simulink model "Trotter_nonsymbolic_VarPhiD"  (R2024a)
settings: Solver=daessc  StartTime=0.0  StopTime=5  FixedStep=1e-5  MaxStep=1e-3  RelTol=1e-5  AbsTol=1e-5  EnableMultiTasking=on
values from neighbouring files (symbols this model uses):
  alpha0 = states{3}(indexVector{3})    [RunAllVPPTrials.m]    (also in SimulationConfig.m = 1.74532925199)
  Bground = 5e3    (= 5000)    [SimulationConfig.m]
  grav = -9.80665    [SimulationConfig.m]
  groundLx = 1000    [SimulationConfig.m]
  groundLy = 1000    [SimulationConfig.m]
  groundThickness = 0.1    [SimulationConfig.m]
  hipSwingStiffness = states{6}(indexVector{6})    [RunAllVPPTrials.m]    (also in SimulationConfig.m = 1000)
  Ka = states{7}(indexVector{7})    [RunAllVPPTrials.m]    (also in SimulationConfig.m = 500)
  Kground = 1e5    (= 100000)    [SimulationConfig.m]
  L1 = 1    [SimulationConfig.m]
  L2 = 1    [SimulationConfig.m]
  m1 = 0.001    [SimulationConfig.m]
  m2 = 0.001    [SimulationConfig.m]
  maxKgLimit = 40000    [SimulationConfig.m]
  mf = 0.001    [SimulationConfig.m]
  mHip = 10    [SimulationConfig.m]
  omega = (strideAngle*pi/180)*(2*hipFreq)    [RunAllVPPTrials.m]    (also in SimulationConfig.m = 2.79252680319)
  phi0 = acos((L1^2-L2^2-f2h0^2)/-(2*L2*f2h0))    [RunAllVPPTrials.m]    (also in SimulationConfig.m)
  rf = 0.05    [SimulationConfig.m]
  shouldIAdaptKp = 1    [RunAllVPPTrials.m]    (also in SimulationConfig.m)
  startingHipStiffness = 1000    [SimulationConfig.m]
  startupTime = 0    [SimulationConfig.m]
  strideAngle = states{4}(indexVector{4})    [RunAllVPPTrials.m]    (also in SimulationConfig.m = 40)
  torsoHeight = 0.2    [SimulationConfig.m]
  torsoLength = 2.5    [SimulationConfig.m]
  torsoWidth = 0.2    [SimulationConfig.m]
  y0 = f2h0*sin(beta0+pi/2)    [RunAllVPPTrials.m]    (also in SimulationConfig.m)
  yOffset = 0.1    [SimulationConfig.m]
undefined symbols (not defined in the file or in its folder): X, Y, Z
libraries: sm_lib x113, nesl_utility x88, Contact_Forces_Lib x16, simulink x8
(part 7 of 7)

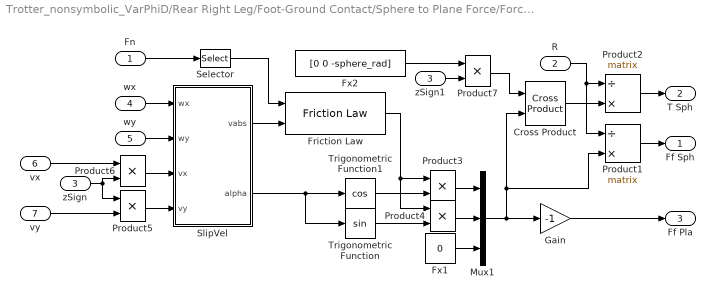
== system Trotter_nonsymbolic_VarPhiD/Rear Right Leg/Foot-Ground Contact/Sphere to Plane Force/Forces/Ff ==
  Fn : Inport
  R : Inport  Port=2
  zSign : Inport  Port=3
  wx : Inport  Port=4
  wy : Inport  Port=5
  vx : Inport  Port=6
  vy : Inport  Port=7
  Cross Product : Contact_Forces_Lib/Math/Cross Product  SystemSampleTime=-1  VariantActivationTime=update diagram  AllowFlexibleInterface=on  Latency=0  AutoFrameSizeCalculation=off
      settings: SourceProductName=Simscape Multibody Contact Forces Library
  Friction Law : Contact_Forces_Lib/Friction Law  SystemSampleTime=-1  LabelModeActiveChoice=Stick_Slip_C  VariantActivationTime=update diagram  AllowFlexibleInterface=on  Latency=0  AutoFrameSizeCalculation=off
      settings: SourceProductName=Simscape Multibody Contact Forces Library
  Fx1 : Constant  Value=0
  Fx2 : Constant  Value=[0 0 -sphere_rad]
  Gain : Gain  Gain=-1
  Mux1 : Mux  Inputs=3
  Product1 : Product  Inputs=/*  Multiplication=Matrix(*)
  Product2 : Product  Inputs=/*  Multiplication=Matrix(*)
  Product{3..7} (5 alike) : Product
  Selector : Selector  InputPortWidth=3  IndexOptions=Index vector (dialog)  Indices=3  OutputSizes=1
  SlipVel : Subsystem
  Trigonometric Function : Trigonometry
  Trigonometric Function1 : Trigonometry  Operator=cos
  zSign1 : InportShadow  Port=3
  Ff Sph : Outport  VectorParamsAs1DForOutWhenUnconnected=off
  T Sph : Outport  Port=2  VectorParamsAs1DForOutWhenUnconnected=off
  Ff Pla : Outport  Port=3  VectorParamsAs1DForOutWhenUnconnected=off
  wires:
  Product7/1 -> Cross Product/1
  zSign1/1 -> Product7/2
  Product6/1 -> SlipVel/3(vx)
  zSign/1 -> Product6/2, Product5/1
  Product5/1 -> SlipVel/4(vy)
  Fx2/1 -> Product7/1
  R/1 -> Product2/1, Product1/1
  Cross Product/1 -> Product2/2
  Product1/1 -> Ff Sph/1
  Mux1/1 -> Product1/2, Cross Product/2, Gain/1
  Product2/1 -> T Sph/1
  vy/1 -> Product5/2
  wy/1 -> SlipVel/2(wy)
  wx/1 -> SlipVel/1(wx)
  vx/1 -> Product6/1
  Trigonometric Function/1 -> Product4/2
  Fx1/1 -> Mux1/3
  Product3/1 -> Mux1/1
  Product4/1 -> Mux1/2
  Friction Law/1 -> Product4/1, Product3/1
  Selector/1 -> Friction Law/1
  SlipVel/1(vabs) -> Friction Law/2
  Trigonometric Function1/1 -> Product3/2
  SlipVel/2(alpha) -> Trigonometric Function1/1, Trigonometric Function/1
  Gain/1 -> Ff Pla/1
  Fn/1 -> Selector/1

== system Trotter_nonsymbolic_VarPhiD/Rear Right Leg/Foot-Ground Contact/Sphere to Plane Force/Forces/Fn ==
  R : Inport
  SprF : Inport  Port=2
  DamF : Inport  Port=3
  Fx : Constant  Value=0
  Gain : Gain  Gain=-1
  Mux : Mux  Inputs=3
  Product2 : Product  Inputs=/*  Multiplication=Matrix(*)
  Sum : Sum
  Fn : Outport  VectorParamsAs1DForOutWhenUnconnected=off
  FnF : Outport  Port=2  VectorParamsAs1DForOutWhenUnconnected=off
  FnB : Outport  Port=3  VectorParamsAs1DForOutWhenUnconnected=off
  wires:
  SprF/1 -> Sum/1
  DamF/1 -> Sum/2
  Sum/1 -> Mux/3, Fn/1
  Fx/1 -> Mux/2, Mux/1
  R/1 -> Product2/1
  Gain/1 -> FnB/1
  Product2/1 -> FnF/1
  Mux/1 -> Product2/2, Gain/1

== system Trotter_nonsymbolic_VarPhiD/Front Left Leg/Foot-Ground Contact/Sphere to Plane Force/Forces/Ff/SlipVel ==
  wx : Inport
  wy : Inport  Port=2
  vx : Inport  Port=3
  vy : Inport  Port=4
  Fx1 : Constant  Value=sphere_rad
  Math Function : Math  Operator=square  SignedPower=on
  Math Function1 : Math  Operator=square  SignedPower=on
  Product3 : Product
  Product4 : Product
  Sqrt : Sqrt
  Sum1 : Sum  Inputs=|++
  Sum2 : Sum  Inputs=|-+
  Sum3 : Sum  Inputs=|++
  Trigonometric Function : Trigonometry  Operator=atan2
  vabs : Outport  VectorParamsAs1DForOutWhenUnconnected=off
  alpha : Outport  Port=2  VectorParamsAs1DForOutWhenUnconnected=off
  wires:
  wx/1 -> Product3/1
  Product3/1 -> Sum1/1
  wy/1 -> Product4/2
  vx/1 -> Sum2/2
  Fx1/1 -> Product3/2, Product4/1
  vy/1 -> Sum1/2
  Product4/1 -> Sum2/1
  Trigonometric Function/1 -> alpha/1
  Sqrt/1 -> vabs/1
  Sum3/1 -> Sqrt/1
  Math Function/1 -> Sum3/1
  Math Function1/1 -> Sum3/2
  Sum1/1 -> Trigonometric Function/1, Math Function/1  "slipy"
  Sum2/1 -> Trigonometric Function/2, Math Function1/1  "slipx"

== system Trotter_nonsymbolic_VarPhiD/Front Right Leg/Foot-Ground Contact/Sphere to Plane Force/Forces/Ff/SlipVel ==
  wx : Inport
  wy : Inport  Port=2
  vx : Inport  Port=3
  vy : Inport  Port=4
  Fx1 : Constant  Value=sphere_rad
  Math Function : Math  Operator=square  SignedPower=on
  Math Function1 : Math  Operator=square  SignedPower=on
  Product3 : Product
  Product4 : Product
  Sqrt : Sqrt
  Sum1 : Sum  Inputs=|++
  Sum2 : Sum  Inputs=|-+
  Sum3 : Sum  Inputs=|++
  Trigonometric Function : Trigonometry  Operator=atan2
  vabs : Outport  VectorParamsAs1DForOutWhenUnconnected=off
  alpha : Outport  Port=2  VectorParamsAs1DForOutWhenUnconnected=off
  wires:
  wx/1 -> Product3/1
  Product3/1 -> Sum1/1
  wy/1 -> Product4/2
  vx/1 -> Sum2/2
  Fx1/1 -> Product3/2, Product4/1
  vy/1 -> Sum1/2
  Product4/1 -> Sum2/1
  Trigonometric Function/1 -> alpha/1
  Sqrt/1 -> vabs/1
  Sum3/1 -> Sqrt/1
  Math Function/1 -> Sum3/1
  Math Function1/1 -> Sum3/2
  Sum1/1 -> Trigonometric Function/1, Math Function/1  "slipy"
  Sum2/1 -> Trigonometric Function/2, Math Function1/1  "slipx"

== system Trotter_nonsymbolic_VarPhiD/Rear Left Leg/Foot-Ground Contact/Sphere to Plane Force/Forces/Ff/SlipVel ==
  wx : Inport
  wy : Inport  Port=2
  vx : Inport  Port=3
  vy : Inport  Port=4
  Fx1 : Constant  Value=sphere_rad
  Math Function : Math  Operator=square  SignedPower=on
  Math Function1 : Math  Operator=square  SignedPower=on
  Product3 : Product
  Product4 : Product
  Sqrt : Sqrt
  Sum1 : Sum  Inputs=|++
  Sum2 : Sum  Inputs=|-+
  Sum3 : Sum  Inputs=|++
  Trigonometric Function : Trigonometry  Operator=atan2
  vabs : Outport  VectorParamsAs1DForOutWhenUnconnected=off
  alpha : Outport  Port=2  VectorParamsAs1DForOutWhenUnconnected=off
  wires:
  wx/1 -> Product3/1
  Product3/1 -> Sum1/1
  wy/1 -> Product4/2
  vx/1 -> Sum2/2
  Fx1/1 -> Product3/2, Product4/1
  vy/1 -> Sum1/2
  Product4/1 -> Sum2/1
  Trigonometric Function/1 -> alpha/1
  Sqrt/1 -> vabs/1
  Sum3/1 -> Sqrt/1
  Math Function/1 -> Sum3/1
  Math Function1/1 -> Sum3/2
  Sum1/1 -> Trigonometric Function/1, Math Function/1  "slipy"
  Sum2/1 -> Trigonometric Function/2, Math Function1/1  "slipx"

== system Trotter_nonsymbolic_VarPhiD/Rear Right Leg/Foot-Ground Contact/Sphere to Plane Force/Forces/Ff/SlipVel ==
  wx : Inport
  wy : Inport  Port=2
  vx : Inport  Port=3
  vy : Inport  Port=4
  Fx1 : Constant  Value=sphere_rad
  Math Function : Math  Operator=square  SignedPower=on
  Math Function1 : Math  Operator=square  SignedPower=on
  Product3 : Product
  Product4 : Product
  Sqrt : Sqrt
  Sum1 : Sum  Inputs=|++
  Sum2 : Sum  Inputs=|-+
  Sum3 : Sum  Inputs=|++
  Trigonometric Function : Trigonometry  Operator=atan2
  vabs : Outport  VectorParamsAs1DForOutWhenUnconnected=off
  alpha : Outport  Port=2  VectorParamsAs1DForOutWhenUnconnected=off
  wires:
  wx/1 -> Product3/1
  Product3/1 -> Sum1/1
  wy/1 -> Product4/2
  vx/1 -> Sum2/2
  Fx1/1 -> Product3/2, Product4/1
  vy/1 -> Sum1/2
  Product4/1 -> Sum2/1
  Trigonometric Function/1 -> alpha/1
  Sqrt/1 -> vabs/1
  Sum3/1 -> Sqrt/1
  Math Function/1 -> Sum3/1
  Math Function1/1 -> Sum3/2
  Sum1/1 -> Trigonometric Function/1, Math Function/1  "slipy"
  Sum2/1 -> Trigonometric Function/2, Math Function1/1  "slipx"

== matlab function Trotter_nonsymbolic_VarPhiD/Left Side Trajectory Generator ==
  data: t input; y_out output; omega parameter; strideAngle parameter; tau output
function [y_out,tau] = fcn(t, omega, strideAngle)
r = (strideAngle*pi/180)/2;% +/- rad (total leg sweep angle is 2*strideAngle)
T = 4*r/omega;
% tau = mod(t+T/4,T)/T; % This starts the trajectory as if the leg is vertically downward during retraction
tau = mod(t+T/2,T)/T; % This starts the trajectory as if the leg is in a backward position a little before protraction begins
% tau = mod(t,T)/T;       % This starts the trajectory as if the leg is in a forward position, right as retraction begins
if tau<0.5
    y_out = r-omega*T*tau;
    dy_out = -omega*T;
else
    y_out = -r - omega*T*(tau-0.5)...
        +(24*r+6*omega*T)*(tau-0.5)^2+(-32*r-8*omega*T)*(tau-0.5)^3;
    dy_out = r*(-96*tau^2+144*tau-48)+(-24*tau^2+36*tau-13)*T*omega;
end

== matlab function Trotter_nonsymbolic_VarPhiD/Front Left Leg/Toe lift ==
  data: tau input; y output; L1 parameter
function y = fcn(tau, L1)
% A = 8*L1;
% y = A*(u-0.75)^2+(1/4)*L1;
% y = min(y,3*L1/4);

a0 = 1/2;
a1 = 0;
a2 = -12;
a3 = 16;
if(tau>=0.5)
    y = L1*(abs((a0+a1*(tau-0.5)+a2*(tau-0.5).^2+a3*(tau-0.5).^3))+0.25);
else
    y = L1*0.75;
end

== matlab function Trotter_nonsymbolic_VarPhiD/Right Side Trajectory Generator ==
  data: t input; y_out output; omega parameter; strideAngle parameter; tau output
function [y_out,tau] = fcn(t, omega, strideAngle)
r = (strideAngle*pi/180)/2;% +/- rad (total leg sweep angle is 2*strideAngle)
T = 4*r/omega;
% tau = mod(t+T/4,T)/T; % This starts the trajectory as if the leg is vertically downward during retraction
% tau = mod(t+T/2,T)/T; % This starts the trajectory as if the leg is in a backward position a little before protraction begins
tau = mod(t,T)/T;       % This starts the trajectory as if the leg is in a forward position, right as retraction begins
if tau<0.5
    y_out = r-omega*T*tau;
    dy_out = -omega*T;
else
    y_out = -r - omega*T*(tau-0.5)...
        +(24*r+6*omega*T)*(tau-0.5)^2+(-32*r-8*omega*T)*(tau-0.5)^3;
    dy_out = r*(-96*tau^2+144*tau-48)+(-24*tau^2+36*tau-13)*T*omega;
end

== matlab function Trotter_nonsymbolic_VarPhiD/Rear Left Leg/Toe lift ==
  data: tau input; y output; L1 parameter
function y = fcn(tau, L1)
% A = 8*L1;
% y = A*(u-0.75)^2+(1/4)*L1;
% y = min(y,3*L1/4);

a0 = 1/2;
a1 = 0;
a2 = -12;
a3 = 16;
if(tau>=0.5)
    y = L1*(abs((a0+a1*(tau-0.5)+a2*(tau-0.5).^2+a3*(tau-0.5).^3))+0.25);
else
    y = L1*0.75;
end

== matlab function Trotter_nonsymbolic_VarPhiD/Front Right Leg/MATLAB Function ==
  data: tau input; y output; L1 parameter
function y = fcn(tau, L1)
% A = 8*L1;
% y = A*(u-0.75)^2+(1/4)*L1;
% y = min(y,3*L1/4);

a0 = 1/2;
a1 = 0;
a2 = -12;
a3 = 16;
if(tau>=0.5)
    y = L1*(abs((a0+a1*(tau-0.5)+a2*(tau-0.5).^2+a3*(tau-0.5).^3))+0.25);
else
    y = L1*0.75;
end

== matlab function Trotter_nonsymbolic_VarPhiD/Front Left Shoulder Joint/Calculate Kg Nonsymbolic ==
  data: time input; phiD input; f2hX input; f2hY input; gammaDesired input; gc input; deltaGamma input; tauHip output; Kout output; startingHipStiffness parameter; hipSwingStiffness parameter; startupTime parameter; shouldIAdaptKp parameter; L1 parameter; L2 parameter; alpha0 parameter; Ka parameter; maxKgLimit parameter
function [tauHip,Kout]  = fcn(time, phiD, f2hX, f2hY, gammaDesired, gc, deltaGamma, startingHipStiffness, hipSwingStiffness, startupTime, shouldIAdaptKp, L1, L2, alpha0, Ka, maxKgLimit)
persistent time_old;
if isempty(time_old)
    time_old = 0;
end
persistent Kg_pers;
if isempty(Kg_pers)
    Kg_pers = 1000;
end

if shouldIAdaptKp==1
    if time>startupTime
        if gc>0
            if time-time_old>=0.001
                x = f2hX;
                y = f2hY;
                gamma0 = gammaDesired+pi/2;
                thetad = phiD;
                Kg_pers = -((Ka*y*(alpha0 + acos((0.5000*L1^2 + 0.5000*L2^2 - 0.5000*x^2 - 0.5000*y^2)/(L1*L2)) - pi))/(L1*L2*(1 - (0.2500*(L1^2 + L2^2 - x^2 - y^2)^2)/(L1^2*L2^2))^0.5000) - (Ka*x*tan(thetad)*(alpha0 + acos((0.5000*L1^2 + 0.5000*L2^2 - 0.5000*x^2 - 0.5000*y^2)/(L1*L2)) - pi))/(L1*L2*(1 - (0.2500*(L1^2 + L2^2 - x^2 - y^2)^2)/(L1^2*L2^2))^0.5000))/((acos((- 0.5000*L1^2 + 0.5000*L2^2 + 0.5000*x^2 + 0.5000*y^2)/(L2*(x^2 + y^2)^0.5000)) + atan2(1*y, x) - gamma0)*(tan(thetad)*((x/(L2*(x^2 + y^2)^0.5000) - (0.5000*x*(- L1^2 + L2^2 + x^2 + y^2))/(L2*(x^2 + y^2)^1.5000))/(1 - (0.2500*(- L1^2 + L2^2 + x^2 + y^2)^2)/(L2^2*(x^2 + y^2)))^0.5000 + y/(x^2 + y^2)) - (y/(L2*(x^2 + y^2)^0.5000) - (0.5000*y*(- L1^2 + L2^2 + x^2 + y^2))/(L2*(x^2 + y^2)^1.5000))/(1 - (0.2500*(- L1^2 + L2^2 + x^2 + y^2)^2)/(L2^2*(x^2 + y^2)))^0.5000 + x/(x^2 + y^2)));
                if ~isreal(Kg_pers)
                    Kg_pers=60;
                end
                Kg_pers = min(max(100,Kg_pers),maxKgLimit);
                time_old = time;
            end
        else
            Kg_pers = hipSwingStiffness;
        end
    else
        Kg_pers = startingHipStiffness;
    end
else
    Kg_pers = hipSwingStiffness;
end
tauHip = Kg_pers*deltaGamma;
Kout = Kg_pers;

% I added pi/2 to gammaDesired because the simulation has gamm=0deg as
% vertical but the matrix calculations and derivations used gamma=0deg as
% horizontal.

== matlab function Trotter_nonsymbolic_VarPhiD/Rear Left Hip Joint/Calculate Kg Nonsymbolic ==
  data: time input; phiD input; f2hX input; f2hY input; gammaDesired input; gc input; deltaGamma input; tauHip output; Kout output; startingHipStiffness parameter; hipSwingStiffness parameter; startupTime parameter; shouldIAdaptKp parameter; L1 parameter; L2 parameter; alpha0 parameter; Ka parameter; maxKgLimit parameter
function [tauHip,Kout]  = fcn(time, phiD, f2hX, f2hY, gammaDesired, gc, deltaGamma, startingHipStiffness, hipSwingStiffness, startupTime, shouldIAdaptKp, L1, L2, alpha0, Ka, maxKgLimit)
persistent time_old;
if isempty(time_old)
    time_old = 0;
end
persistent Kg_pers;
if isempty(Kg_pers)
    Kg_pers = 1000;
end

if shouldIAdaptKp==1
    if time>startupTime
        if gc>0
            if time-time_old>=0.001
                x = f2hX;
                y = f2hY;
                gamma0 = gammaDesired+pi/2;
                thetad = phiD;
                Kg_pers = -((Ka*y*(alpha0 + acos((0.5000*L1^2 + 0.5000*L2^2 - 0.5000*x^2 - 0.5000*y^2)/(L1*L2)) - pi))/(L1*L2*(1 - (0.2500*(L1^2 + L2^2 - x^2 - y^2)^2)/(L1^2*L2^2))^0.5000) - (Ka*x*tan(thetad)*(alpha0 + acos((0.5000*L1^2 + 0.5000*L2^2 - 0.5000*x^2 - 0.5000*y^2)/(L1*L2)) - pi))/(L1*L2*(1 - (0.2500*(L1^2 + L2^2 - x^2 - y^2)^2)/(L1^2*L2^2))^0.5000))/((acos((- 0.5000*L1^2 + 0.5000*L2^2 + 0.5000*x^2 + 0.5000*y^2)/(L2*(x^2 + y^2)^0.5000)) + atan2(1*y, x) - gamma0)*(tan(thetad)*((x/(L2*(x^2 + y^2)^0.5000) - (0.5000*x*(- L1^2 + L2^2 + x^2 + y^2))/(L2*(x^2 + y^2)^1.5000))/(1 - (0.2500*(- L1^2 + L2^2 + x^2 + y^2)^2)/(L2^2*(x^2 + y^2)))^0.5000 + y/(x^2 + y^2)) - (y/(L2*(x^2 + y^2)^0.5000) - (0.5000*y*(- L1^2 + L2^2 + x^2 + y^2))/(L2*(x^2 + y^2)^1.5000))/(1 - (0.2500*(- L1^2 + L2^2 + x^2 + y^2)^2)/(L2^2*(x^2 + y^2)))^0.5000 + x/(x^2 + y^2)));
                if ~isreal(Kg_pers)
                    Kg_pers=60;
                end
                Kg_pers = min(max(100,Kg_pers),maxKgLimit);
                time_old = time;
            end
        else
            Kg_pers = hipSwingStiffness;
        end
    else
        Kg_pers = startingHipStiffness;
    end
else
    Kg_pers = hipSwingStiffness;
end
tauHip = Kg_pers*deltaGamma;
Kout = Kg_pers;

% I added pi/2 to gammaDesired because the simulation has gamm=0deg as
% vertical but the matrix calculations and derivations used gamma=0deg as
% horizontal.

== matlab function Trotter_nonsymbolic_VarPhiD/Rear Left Leg/Foot to COM Angle Generator ==
  data: x input; f2COMAngle output; z input
function f2COMAngle = fcn(x,z)

f2COMAngle = atan2(z,x);

% Ok, this is for the front right leg, which is pointed backwards as
% compared to how the model is defined for the leg equation. An angle of
% 120 points in between the knee and hip for the front legs, but in the
% original equation I defined the angles between the knee and hip to be
% less than 90 degrees. So I want to convert an angle like 120 into an
% angle like 60. So the equation I want is 90-(120-90) which is actually
% 180-120 so since im using radians I did pi - atan() to give me my final
% value for the front leg.

== matlab function Trotter_nonsymbolic_VarPhiD/Front Right Leg/Foot to COM Angle Generator ==
  data: x input; f2COMAngle output; z input
function f2COMAngle = fcn(x,z)

f2COMAngle = pi-atan2(z,x);

% Ok, this is for the front right leg, which is pointed backwards as
% compared to how the model is defined for the leg equation. An angle of
% 120 points in between the knee and hip for the front legs, but in the
% original equation I defined the angles between the knee and hip to be
% less than 90 degrees. So I want to convert an angle like 120 into an
% angle like 60. So the equation I want is 90-(120-90) which is actually
% 180-120 so since im using radians I did pi - atan() to give me my final
% value for the front leg.

== matlab function Trotter_nonsymbolic_VarPhiD/Front Left Leg/Foot to COM Angle Generator ==
  data: x input; f2COMAngle output; z input
function f2COMAngle = fcn(x,z)

f2COMAngle = pi-atan2(z,x);

% Ok, this is for the front right leg, which is pointed backwards as
% compared to how the model is defined for the leg equation. An angle of
% 120 points in between the knee and hip for the front legs, but in the
% original equation I defined the angles between the knee and hip to be
% less than 90 degrees. So I want to convert an angle like 120 into an
% angle like 60. So the equation I want is 90-(120-90) which is actually
% 180-120 so since im using radians I did pi - atan() to give me my final
% value for the front leg.

== matlab function Trotter_nonsymbolic_VarPhiD/Front Right Shoulder Joint/Calculate Kp with Natural phiD Profile ==
  data: time input; phiD input; f2hX input; f2hY input; gammaDesired input; gc input; deltaGamma input; tauHip output; Kout output; hipSwingStiffness parameter; shouldIAdaptKp parameter; L1 parameter; L2 parameter; alpha0 parameter; Ka parameter; maxKgLimit parameter; rawKout output; startingHipStiffness parameter; startupTime parameter
function [tauHip,Kout,rawKout]  = fcn(time, phiD, f2hX, f2hY, gammaDesired, gc, deltaGamma, hipSwingStiffness, shouldIAdaptKp, L1, L2, alpha0, Ka, maxKgLimit, startingHipStiffness, startupTime)
persistent time_old;
if isempty(time_old)
    time_old = 0;
end
persistent Kg_pers;
if isempty(Kg_pers)
    Kg_pers = 1000;
end
persistent rawKg;
if isempty(rawKg)
    rawKg = 1000;
end

if shouldIAdaptKp==1
    if time>startupTime
        if gc>0
            if time-time_old>=0.001
                x = f2hX;
                y = f2hY;
                gamma0 = gammaDesired+pi/2;
                thetad = phiD*pi/180;
                if phiD==0
                    Kg_pers = hipSwingStiffness;
                else
                    Kg_pers = -((Ka*y*(alpha0 + acos((0.5000*L1^2 + 0.5000*L2^2 - 0.5000*x^2 - 0.5000*y^2)/(L1*L2)) - pi))/(L1*L2*(1 - (0.2500*(L1^2 + L2^2 - x^2 - y^2)^2)/(L1^2*L2^2))^0.5000) - (Ka*x*tan(thetad)*(alpha0 + acos((0.5000*L1^2 + 0.5000*L2^2 - 0.5000*x^2 - 0.5000*y^2)/(L1*L2)) - pi))/(L1*L2*(1 - (0.2500*(L1^2 + L2^2 - x^2 - y^2)^2)/(L1^2*L2^2))^0.5000))/((acos((- 0.5000*L1^2 + 0.5000*L2^2 + 0.5000*x^2 + 0.5000*y^2)/(L2*(x^2 + y^2)^0.5000)) + atan2(1*y, x) - gamma0)*(tan(thetad)*((x/(L2*(x^2 + y^2)^0.5000) - (0.5000*x*(- L1^2 + L2^2 + x^2 + y^2))/(L2*(x^2 + y^2)^1.5000))/(1 - (0.2500*(- L1^2 + L2^2 + x^2 + y^2)^2)/(L2^2*(x^2 + y^2)))^0.5000 + y/(x^2 + y^2)) - (y/(L2*(x^2 + y^2)^0.5000) - (0.5000*y*(- L1^2 + L2^2 + x^2 + y^2))/(L2*(x^2 + y^2)^1.5000))/(1 - (0.2500*(- L1^2 + L2^2 + x^2 + y^2)^2)/(L2^2*(x^2 + y^2)))^0.5000 + x/(x^2 + y^2)));
                end
                if ~isreal(Kg_pers)
                    Kg_pers=101;
                end
                rawKg = Kg_pers;
                Kg_pers = min(max(100,Kg_pers),maxKgLimit);
                time_old = time;
            end
        else
            Kg_pers = hipSwingStiffness;
            rawKg = Kg_pers;
        end
    else
        Kg_pers = startingHipStiffness;
        rawKg = Kg_pers;
    end
else
    Kg_pers = hipSwingStiffness;
    rawKg = Kg_pers;
end
tauHip = Kg_pers*deltaGamma;
Kout = Kg_pers;
rawKout = rawKg;

% I added pi/2 to gammaDesired because the simulation has gamm=0deg as
% vertical but the matrix calculations and derivations used gamma=0deg as
% horizontal.

== matlab function Trotter_nonsymbolic_VarPhiD/Rear Right Hip Joint/Calculate Kg Nonsymbolic ==
  data: time input; phiD input; f2hX input; f2hY input; gammaDesired input; gc input; deltaGamma input; tauHip output; Kout output; startingHipStiffness parameter; hipSwingStiffness parameter; startupTime parameter; shouldIAdaptKp parameter; L1 parameter; L2 parameter; alpha0 parameter; Ka parameter; maxKgLimit parameter
function [tauHip,Kout]  = fcn(time, phiD, f2hX, f2hY, gammaDesired, gc, deltaGamma, startingHipStiffness, hipSwingStiffness, startupTime, shouldIAdaptKp, L1, L2, alpha0, Ka, maxKgLimit)
persistent time_old;
if isempty(time_old)
    time_old = 0;
end
persistent Kg_pers;
if isempty(Kg_pers)
    Kg_pers = 1000;
end

if shouldIAdaptKp==1
    if time>startupTime
        if gc>0
            if time-time_old>=0.001
                x = f2hX;
                y = f2hY;
                gamma0 = gammaDesired+pi/2;
                thetad = phiD;
                Kg_pers = -((Ka*y*(alpha0 + acos((0.5000*L1^2 + 0.5000*L2^2 - 0.5000*x^2 - 0.5000*y^2)/(L1*L2)) - pi))/(L1*L2*(1 - (0.2500*(L1^2 + L2^2 - x^2 - y^2)^2)/(L1^2*L2^2))^0.5000) - (Ka*x*tan(thetad)*(alpha0 + acos((0.5000*L1^2 + 0.5000*L2^2 - 0.5000*x^2 - 0.5000*y^2)/(L1*L2)) - pi))/(L1*L2*(1 - (0.2500*(L1^2 + L2^2 - x^2 - y^2)^2)/(L1^2*L2^2))^0.5000))/((acos((- 0.5000*L1^2 + 0.5000*L2^2 + 0.5000*x^2 + 0.5000*y^2)/(L2*(x^2 + y^2)^0.5000)) + atan2(1*y, x) - gamma0)*(tan(thetad)*((x/(L2*(x^2 + y^2)^0.5000) - (0.5000*x*(- L1^2 + L2^2 + x^2 + y^2))/(L2*(x^2 + y^2)^1.5000))/(1 - (0.2500*(- L1^2 + L2^2 + x^2 + y^2)^2)/(L2^2*(x^2 + y^2)))^0.5000 + y/(x^2 + y^2)) - (y/(L2*(x^2 + y^2)^0.5000) - (0.5000*y*(- L1^2 + L2^2 + x^2 + y^2))/(L2*(x^2 + y^2)^1.5000))/(1 - (0.2500*(- L1^2 + L2^2 + x^2 + y^2)^2)/(L2^2*(x^2 + y^2)))^0.5000 + x/(x^2 + y^2)));
                if ~isreal(Kg_pers)
                    Kg_pers=60;
                end
                Kg_pers = min(max(100,Kg_pers),maxKgLimit);
                time_old = time;
            end
        else
            Kg_pers = hipSwingStiffness;
        end
    else
        Kg_pers = startingHipStiffness;
    end
else
    Kg_pers = hipSwingStiffness;
end
tauHip = Kg_pers*deltaGamma;
Kout = Kg_pers;

% I added pi/2 to gammaDesired because the simulation has gamm=0deg as
% vertical but the matrix calculations and derivations used gamma=0deg as
% horizontal.

== matlab function Trotter_nonsymbolic_VarPhiD/Rear Right Leg/Toe lift ==
  data: tau input; y output; L1 parameter
function y = fcn(tau, L1)
% This function defines the trajectory of the toe lift movement during the
% swing phase of this foot based on tau which comes from the desired hip
% trajectory generator
a0 = 1/2;
a1 = 0;
a2 = -12;
a3 = 16;
if(tau>=0.5)
    y = L1*(abs((a0+a1*(tau-0.5)+a2*(tau-0.5).^2+a3*(tau-0.5).^3))+0.25);
else
    y = L1*0.75;
end

== matlab function Trotter_nonsymbolic_VarPhiD/Rear Right Leg/Foot to COM Angle Generator ==
  data: x input; f2COMAngle output; z input
function f2COMAngle = fcn(x,z)

f2COMAngle = atan2(z,x);

% Ok, this is for the front right leg, which is pointed backwards as
% compared to how the model is defined for the leg equation. An angle of
% 120 points in between the knee and hip for the front legs, but in the
% original equation I defined the angles between the knee and hip to be
% less than 90 degrees. So I want to convert an angle like 120 into an
% angle like 60. So the equation I want is 90-(120-90) which is actually
% 180-120 so since im using radians I did pi - atan() to give me my final
% value for the front leg.
